simulink model "LKARefMdl"  (R2025b)
settings: Solver=FixedStepDiscrete  StartTime=0.0  StopTime=inf  FixedStep=Ts  RelTol=1e-3
values from neighbouring files (symbols this model uses):
  PredictionHorizon = 30    [helperLKASetUp.m]
  Ts = 0.1/2    (= 0.05)    [helperLKASetUp.m]
libraries: simulink x4, simulink_extras x1, mpcadaslib x1
settings Model: Creator=The MathWorks, Inc.  LastModifiedBy=diogo
settings SolverCC: AlgebraicLoopSolver=TrustRegion
settings DataIOCC: SaveOutput=off  SaveTime=off  ReturnWorkspaceOutputs=off
settings OptimizationCC: DefaultParameterBehavior=Inlined  UseFloatMulNetSlope=on  DefaultUnderspecifiedDataType=single  UseSpecifiedMinMax=on  InlineInvariantSignals=on  EnhancedBackFolding=on  StrengthReduction=on  PassReuseOutputArgsAs=Individual arguments  ZeroExternalMemoryAtStartup=off  ZeroInternalMemoryAtStartup=off  NoFixptDivByZeroProtection=on  EfficientFloat2IntCast=on  OptimizeBlockOrder=speed  DifferentSizesBufferReuse=on  EfficientTunableParamExpr=on
settings DebuggingCC: ParameterPrecisionLossMsg=none  ParameterTunabilityLossMsg=error  UnconnectedInputMsg=warning  UnconnectedOutputMsg=warning  UnconnectedLineMsg=warning  ArithmeticOperatorsInVariantConditions=warning
settings HardwareCC: ProdLongLongMode=on
settings ModelReferenceCC: EnableRefExpFcnMdlSchedulingChecks=on
settings SFSimCC: SimUseLocalCustomCode=off  MATLABDynamicMemAlloc=off  CustomCodeUndefinedFunction=UseInterfaceOnly  SimTargetLang=C++  SimDLTargetLibrary=mkl-dnn
settings RTWCC: SystemTargetFile=ert.tlc  TemplateMakefile=ert_default_tmf  GenerateReport=on  RTWUseLocalCustomCode=off  BuildConfiguration=Faster Runs  IncludeHyperlinkInReport=on  LaunchReport=on  TargetLang=C++  GenerateTraceInfo=on  GenerateTraceReport=on  GenerateTraceReportSl=on  GenerateTraceReportSf=on  GenerateTraceReportEml=on  GPUComputeCapability=3.5  DLArmComputeVersion=19.05  Description=Embedded Coder
settings CodeAppCC: ForceParamTrailComments=on  IgnoreCustomStorageClasses=off  OperatorAnnotations=on  SimulinkDataObjDesc=on  SFDataObjDesc=on  InsertBlockDesc=on
settings ERTTargetCC: RootIOFormat=Structure reference  ERTCustomFileTemplate=example_file_process.tlc  DynamicArrayContainerType=coder::array  TargetLangStandard=C++03 (ISO)  GenerateSampleERTMain=on  CombineSignalStateStructs=on  SuppressErrorStatus=on  CodeInterfacePackaging=C++ class  SubcomponentCodeInterfacePackaging=C++ class

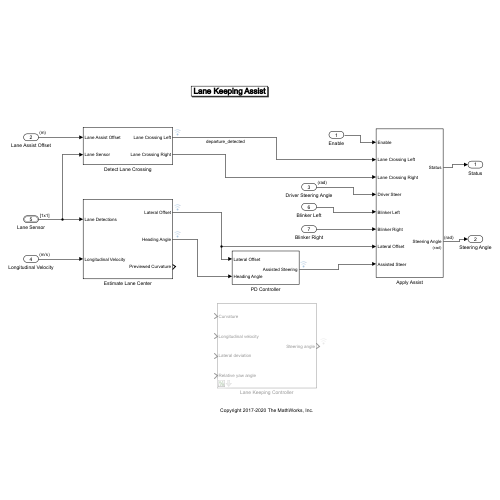
[thumbnail: Simulink's stored preview of the top-level diagram]
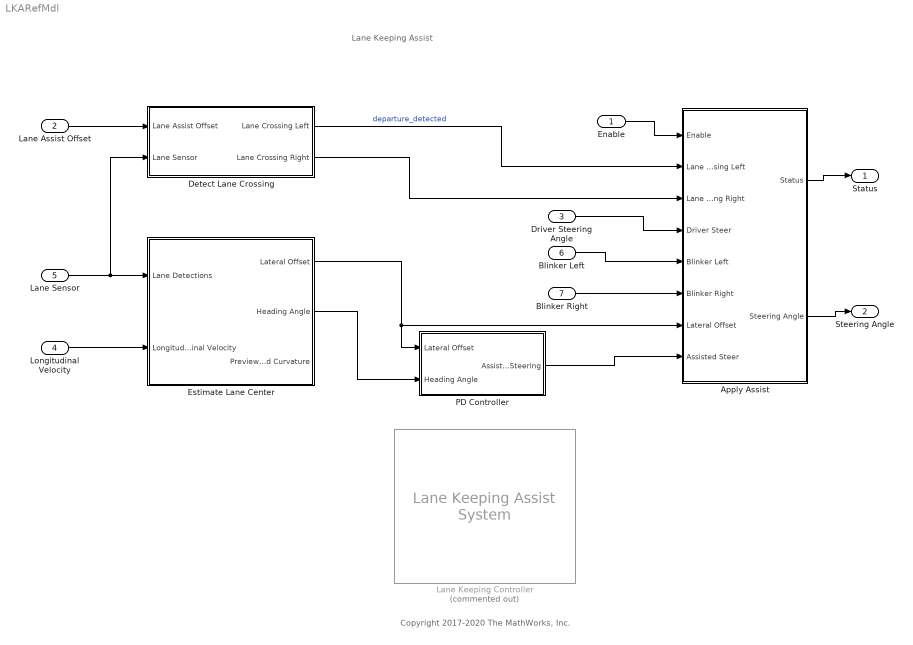
== system LKARefMdl ==
  note: Copyright 2017-2020 The MathWorks, Inc.
  note: Lane Keeping Assist
  Enable : Inport  OutDataTypeStr=boolean  SampleTime=Ts
  Lane Assist Offset : Inport  Port=2  OutDataTypeStr=single  Unit=m  SampleTime=Ts
  Driver Steering Angle : Inport  Port=3  Unit=rad
  Longitudinal Velocity : Inport  Port=4  OutDataTypeStr=single  Unit=m/s  SampleTime=Ts
  Lane Sensor : Inport  Port=5  OutDataTypeStr=Bus: LaneSensor  PortDimensions=[1 1]  SampleTime=Ts  BusOutputAsStruct=on
  Blinker Left : Inport  Port=6
  Blinker Right : Inport  Port=7
  Apply Assist : Subsystem
  Detect Lane Crossing : Subsystem
  Estimate Lane Center : Subsystem  VariantControl=v2
  Lane Keeping Controller : mpcadaslib/Lane Keeping Assist System  Commented=on  ModelType=Use vehicle parameters  VehicleMass=m  VehicleYawInertia=Iz  LengthToFront=lf  LengthToRear=lr  FrontTireStiffness=Cf  RearTireStiffness=Cr  EgoModelMatrixA=[-4.4021 ,-12.4603;1.3913,-5.1868]  EgoModelMatrixB=[24.1270;15.8609]  EgoModelMatrixC=[1,0;0,1]  InitialLongVel=v0_ego  TransportLag=0  MinSteering=-0.5  umin_ext=off  MaxSteering=0.5  umax_ext=off  Ts=Ts  PredictionHorizon=PredictionHorizon  ControllerBehavior=0.200  suboptimal=off  maxiter=10  datatypeopt=single  optmode=off  trackmode=off
  PD Controller : Subsystem
  Status : Outport  PortDimensions=1  VectorParamsAs1DForOutWhenUnconnected=off
  Steering Angle : Outport  Port=2  PortDimensions=1  VectorParamsAs1DForOutWhenUnconnected=off
  wires:
  Lane Assist Offset/1 -> Detect Lane Crossing/1(Lane Assist Offset)
  Driver Steering Angle/1 -> Apply Assist/4(Driver Steer)
  Enable/1 -> Apply Assist/1(Enable)
  Apply Assist/1(Status) -> Status/1
  Apply Assist/2(Steering Angle) -> Steering Angle/1
  Detect Lane Crossing/1(Lane Crossing Left) -> Apply Assist/2(Lane Crossing Left)  "departure_detected"
  Longitudinal Velocity/1 -> Estimate Lane Center/2(Longitudinal Velocity)
  Lane Sensor/1 -> Detect Lane Crossing/2(Lane Sensor), Estimate Lane Center/1(Lane Detections)
  Estimate Lane Center/1(Lateral Offset) -> PD Controller/1(Lateral Offset), Apply Assist/7(Lateral Offset)
  Estimate Lane Center/2(Heading Angle) -> PD Controller/2(Heading Angle)
  PD Controller/1(Assisted Steering) -> Apply Assist/8(Assisted Steer)
  Blinker Left/1 -> Apply Assist/5(Blinker Left)
  Detect Lane Crossing/2(Lane Crossing Right) -> Apply Assist/3(Lane Crossing Right)
  Blinker Right/1 -> Apply Assist/6(Blinker Right)

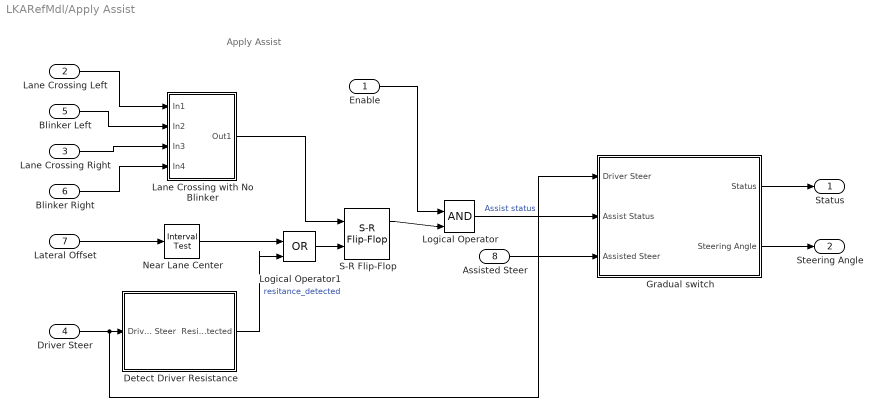
== system LKARefMdl/Apply Assist ==
  note: Apply Assist
  Enable : Inport
  Lane Crossing Left : Inport  Port=2
  Lane Crossing Right : Inport  Port=3
  Driver Steer : Inport  Port=4
  Blinker Left : Inport  Port=5
  Blinker Right : Inport  Port=6
  Lateral Offset : Inport  Port=7
  Assisted Steer : Inport  Port=8
  "Detect Driver Resistance " : Subsystem
  Gradual switch : Subsystem
  Lane Crossing with No Blinker : Subsystem
  Logical Operator : Logic  IconShape=distinctive  AllPortsSameDT=off  OutDataTypeStr=boolean
  Logical Operator1 : Logic  Operator=OR  IconShape=distinctive  AllPortsSameDT=off  OutDataTypeStr=boolean
  Near Lane Center : simulink/Logic and Bit Operations/Interval Test  IntervalClosedRight=on  uplimit=0.1  IntervalClosedLeft=on  lowlimit=-0.1  OutDataTypeStr=boolean
  S-R Flip-Flop : simulink_extras/Flip Flops/S-R Flip-Flop  initial_condition=0
  Status : Outport  VectorParamsAs1DForOutWhenUnconnected=off
  Steering Angle : Outport  Port=2  Unit=rad  VectorParamsAs1DForOutWhenUnconnected=off
  wires:
  Enable/1 -> Logical Operator/1
  Logical Operator/1 -> Gradual switch/2(Assist Status)  "Assist status"
  Driver Steer/1 -> "Detect Driver Resistance "/1(Driver Steer), Gradual switch/1(Driver Steer)
  Gradual switch/1(Status) -> Status/1
  Gradual switch/2(Steering Angle) -> Steering Angle/1
  S-R Flip-Flop/1 -> Logical Operator/2
  Lane Crossing Left/1 -> Lane Crossing with No Blinker/1(In1)
  Blinker Left/1 -> Lane Crossing with No Blinker/2(In2)
  Lane Crossing Right/1 -> Lane Crossing with No Blinker/3(In3)
  Blinker Right/1 -> Lane Crossing with No Blinker/4(In4)
  Lane Crossing with No Blinker/1(Out1) -> S-R Flip-Flop/1
  Near Lane Center/1 -> Logical Operator1/1
  Lateral Offset/1 -> Near Lane Center/1
  "Detect Driver Resistance "/1(Resistance Detected) -> Logical Operator1/2  "resitance_detected"
  Logical Operator1/1 -> S-R Flip-Flop/2
  Assisted Steer/1 -> Gradual switch/3(Assisted Steer)

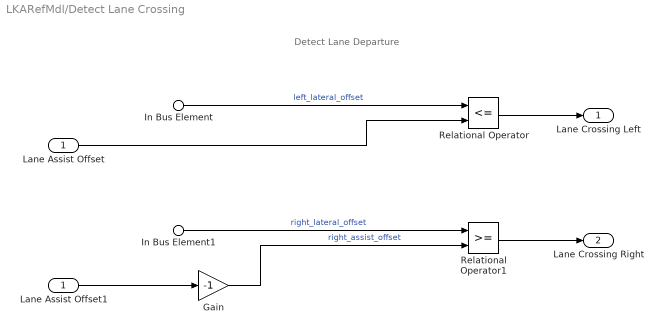
== system LKARefMdl/Detect Lane Crossing ==
  note: Detect Lane Departure
  Lane Assist Offset : Inport
  In Bus Element : Inport  Port=2  PortName=Lane Sensor  Element=Left.LateralOffset
  In Bus Element1 : Inport  Port=2  PortName=Lane Sensor  Element=Right.LateralOffset
  Gain : Gain  Gain=-1
  Lane Assist Offset1 : InportShadow
  Relational Operator : RelationalOperator  Operator=<=  OutDataTypeStr=boolean  RndMeth=Simplest  InputSameDT=off
  Relational Operator1 : RelationalOperator  OutDataTypeStr=boolean  RndMeth=Simplest  InputSameDT=off
  Lane Crossing Left : Outport  VectorParamsAs1DForOutWhenUnconnected=off
  Lane Crossing Right : Outport  Port=2  VectorParamsAs1DForOutWhenUnconnected=off
  wires:
  Lane Assist Offset/1 -> Relational Operator/2
  In Bus Element/1 -> Relational Operator/1  "left_lateral_offset"
  Lane Assist Offset1/1 -> Gain/1
  In Bus Element1/1 -> Relational Operator1/1  "right_lateral_offset"
  Gain/1 -> Relational Operator1/2  "right_assist_offset"
  Relational Operator1/1 -> Lane Crossing Right/1
  Relational Operator/1 -> Lane Crossing Left/1

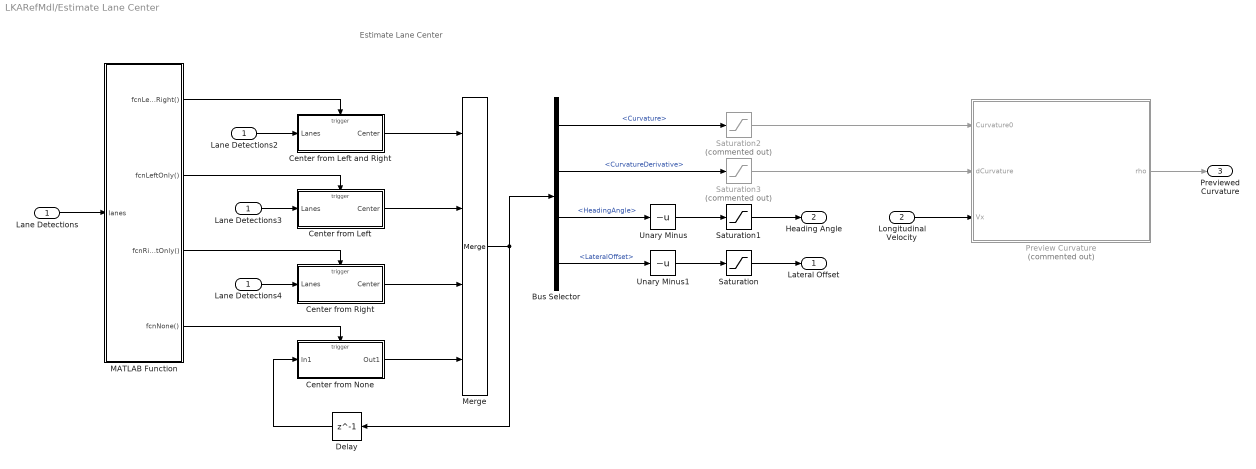
== system LKARefMdl/Estimate Lane Center ==
  note: Estimate Lane Center
  Lane Detections : Inport
  Longitudinal Velocity : Inport  Port=2  OutDataTypeStr=single
  Bus Selector : BusSelector  OutputSignals=Curvature,CurvatureDerivative,HeadingAngle,LateralOffset
  Center from Left : Subsystem  TreatAsAtomicUnit=on
  Center from Left and Right : Subsystem  TreatAsAtomicUnit=on
  Center from None : Subsystem  TreatAsAtomicUnit=on
  Center from Right : Subsystem  TreatAsAtomicUnit=on
  Delay : Delay  DelayLength=1
  Lane Detections2 : InportShadow
  Lane Detections3 : InportShadow
  Lane Detections4 : InportShadow
  MATLAB Function : MATLAB Function  TreatAsAtomicUnit=on
  Merge : Merge  Inputs=4
  Preview Curvature : MATLAB Function  Commented=on  TreatAsAtomicUnit=on  SystemSampleTime=Ts
  Saturation : Saturate
  Saturation1 : Saturate  UpperLimit=0.6  LowerLimit=-0.6
  Saturation2 : Saturate  Commented=on  UpperLimit=0.15  LowerLimit=-0.15
  Saturation3 : Saturate  Commented=on  UpperLimit=0.06  LowerLimit=-0.06
  Unary Minus : UnaryMinus
  Unary Minus1 : UnaryMinus
  Lateral Offset : Outport  VectorParamsAs1DForOutWhenUnconnected=off
  Heading Angle : Outport  Port=2  VectorParamsAs1DForOutWhenUnconnected=off
  Previewed Curvature : Outport  Port=3  VectorParamsAs1DForOutWhenUnconnected=off
  wires:
  Bus Selector/3 -> Unary Minus/1  "<HeadingAngle>"
  Bus Selector/4 -> Unary Minus1/1  "<LateralOffset>"
  Unary Minus1/1 -> Saturation/1
  Longitudinal Velocity/1 -> Preview Curvature/3(Vx)
  Unary Minus/1 -> Saturation1/1
  Saturation/1 -> Lateral Offset/1
  Saturation1/1 -> Heading Angle/1
  Merge/1 -> Delay/1, Bus Selector/1
  Center from Left/1(Center) -> Merge/2
  MATLAB Function/4(fcnNone()) -> Center from None/Trigger
  MATLAB Function/3(fcnRightOnly()) -> Center from Right/Trigger
  Lane Detections2/1 -> Center from Left and Right/1(Lanes)
  Lane Detections/1 -> MATLAB Function/1(lanes)
  Center from Left and Right/1(Center) -> Merge/1
  Delay/1 -> Center from None/1(In1)
  MATLAB Function/1(fcnLeftAndRight()) -> Center from Left and Right/Trigger
  Center from None/1(Out1) -> Merge/4
  MATLAB Function/2(fcnLeftOnly()) -> Center from Left/Trigger
  Lane Detections4/1 -> Center from Right/1(Lanes)
  Lane Detections3/1 -> Center from Left/1(Lanes)
  Center from Right/1(Center) -> Merge/3
  Bus Selector/2 -> Saturation3/1  "<CurvatureDerivative>"
  Preview Curvature/1(rho) -> Previewed Curvature/1
  Saturation3/1 -> Preview Curvature/2(dCurvature)
  Saturation2/1 -> Preview Curvature/1(Curvature0)
  Bus Selector/1 -> Saturation2/1  "<Curvature>"

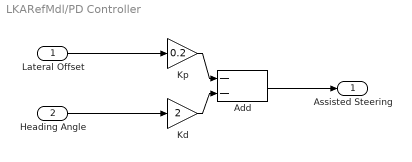
== system LKARefMdl/PD Controller ==
  Lateral Offset : Inport
  Heading Angle : Inport  Port=2
  Add : Sum  Inputs=--
  Kd : Gain  Gain=2
  Kp : Gain  Gain=0.2
  Assisted Steering : Outport
  wires:
  Kp/1 -> Add/1
  Add/1 -> Assisted Steering/1
  Kd/1 -> Add/2
  Heading Angle/1 -> Kd/1
  Lateral Offset/1 -> Kp/1

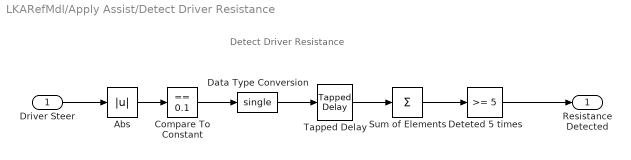
== system LKARefMdl/Apply Assist/Detect Driver Resistance  ==
  note: Detect Driver Resistance
  Driver Steer : Inport
  Abs : Abs  SaturateOnIntegerOverflow=off
  Compare To Constant : simulink/Logic and Bit Operations/Compare To Constant  relop===  const=0.1  OutDataTypeStr=boolean
  Data Type Conversion : DataTypeConversion  OutDataTypeStr=single  SaturateOnIntegerOverflow=off  RndMeth=Floor
  Deteted 5 times : simulink/Logic and Bit Operations/Compare To Constant  relop=>=  const=5  OutDataTypeStr=boolean
  Sum of Elements : Sum  Inputs=+
  Tapped Delay : simulink/Discrete/Tapped Delay  vinit=0.0  samptime=-1  NumDelays=5  DelayOrder=Oldest  includeCurrent=off
  Resistance Detected : Outport  VectorParamsAs1DForOutWhenUnconnected=off
  wires:
  Driver Steer/1 -> Abs/1
  Deteted 5 times/1 -> Resistance Detected/1
  Data Type Conversion/1 -> Tapped Delay/1
  Tapped Delay/1 -> Sum of Elements/1
  Sum of Elements/1 -> Deteted 5 times/1
  Abs/1 -> Compare To Constant/1
  Compare To Constant/1 -> Data Type Conversion/1

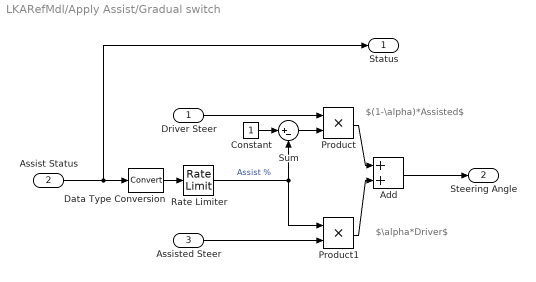
== system LKARefMdl/Apply Assist/Gradual switch ==
  note: $\alpha*Driver$
  note: $(1-\alpha)*Assisted$
  Driver Steer : Inport
  Assist Status : Inport  Port=2
  Assisted Steer : Inport  Port=3
  Add : Sum
  Constant : Constant
  Data Type Conversion : DataTypeConversion  SaturateOnIntegerOverflow=off  RndMeth=Floor
  Product : Product
  Product1 : Product
  Rate Limiter : RateLimiter  RisingSlewLimit=0.25  FallingSlewLimit=-0.25  SampleTimeMode=inherited
  Sum : Sum  Inputs=|+-
  Status : Outport  VectorParamsAs1DForOutWhenUnconnected=off
  Steering Angle : Outport  Port=2  Unit=rad  VectorParamsAs1DForOutWhenUnconnected=off
  wires:
  Rate Limiter/1 -> Product1/1, Sum/2  "Assist %"
  Product/1 -> Add/1
  Assist Status/1 -> Status/1, Data Type Conversion/1
  Constant/1 -> Sum/1
  Add/1 -> Steering Angle/1
  Sum/1 -> Product/2
  Assisted Steer/1 -> Product1/2
  Product1/1 -> Add/2
  Driver Steer/1 -> Product/1
  Data Type Conversion/1 -> Rate Limiter/1

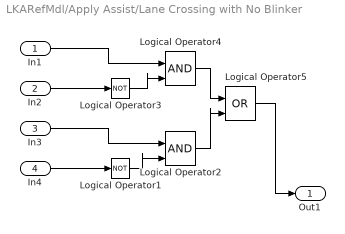
== system LKARefMdl/Apply Assist/Lane Crossing with No Blinker ==
  In1 : Inport
  In2 : Inport  Port=2
  In3 : Inport  Port=3
  In4 : Inport  Port=4
  Logical Operator1 : Logic  Operator=NOT  IconShape=distinctive  AllPortsSameDT=off  OutDataTypeStr=boolean
  Logical Operator2 : Logic  IconShape=distinctive  AllPortsSameDT=off  OutDataTypeStr=boolean
  Logical Operator3 : Logic  Operator=NOT  IconShape=distinctive  AllPortsSameDT=off  OutDataTypeStr=boolean
  Logical Operator4 : Logic  IconShape=distinctive  AllPortsSameDT=off  OutDataTypeStr=boolean
  Logical Operator5 : Logic  Operator=OR  IconShape=distinctive  AllPortsSameDT=off  OutDataTypeStr=boolean
  Out1 : Outport
  wires:
  Logical Operator4/1 -> Logical Operator5/1
  Logical Operator2/1 -> Logical Operator5/2
  Logical Operator3/1 -> Logical Operator4/2
  In2/1 -> Logical Operator3/1
  Logical Operator5/1 -> Out1/1
  In4/1 -> Logical Operator1/1
  Logical Operator1/1 -> Logical Operator2/2
  In3/1 -> Logical Operator2/1
  In1/1 -> Logical Operator4/1

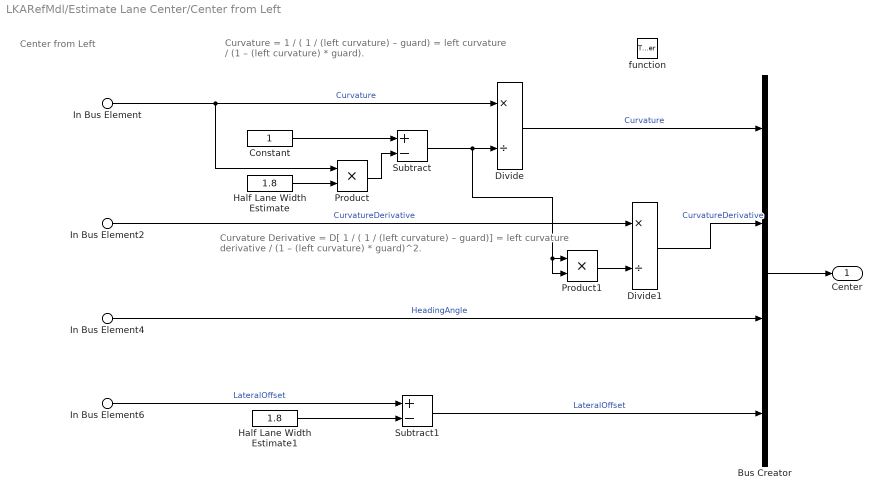
== system LKARefMdl/Estimate Lane Center/Center from Left ==
  note: Curvature
      | = 1 / ( 1 / (left curvature) – guard)
      | = left curvature / (1 – (left curvature) * guard).
  note: Center from Left
  note: Curvature Derivative
      | = D[ 1 / ( 1 / (left curvature) – guard)]
      | = left curvature derivative / (1 – (left curvature) * guard)^2.
  In Bus Element : Inport  PortName=Lanes  Element=Left.Curvature
  In Bus Element2 : Inport  PortName=Lanes  Element=Left.CurvatureDerivative
  In Bus Element4 : Inport  PortName=Lanes  Element=Left.HeadingAngle
  In Bus Element6 : Inport  PortName=Lanes  Element=Left.LateralOffset
  function : TriggerPort  TriggerType=function-call  VariantControl=Variant
  Bus Creator : BusCreator  Inputs=4
  Constant : Constant  OutDataTypeStr=Inherit: Inherit via back propagation
  Divide : Product  Inputs=*/
  Divide1 : Product  Inputs=*/
  Half Lane Width Estimate : Constant  Value=1.8  OutDataTypeStr=Inherit: Inherit via back propagation
  Half Lane Width Estimate1 : Constant  Value=1.8  OutDataTypeStr=Inherit: Inherit via back propagation
  Product : Product
  Product1 : Product
  Subtract : Sum  Inputs=+-
  Subtract1 : Sum  Inputs=+-
  Center : Outport  VectorParamsAs1DForOutWhenUnconnected=off
  wires:
  Bus Creator/1 -> Center/1
  Divide1/1 -> Bus Creator/2  "CurvatureDerivative"
  Divide/1 -> Bus Creator/1  "Curvature"
  In Bus Element4/1 -> Bus Creator/3  "HeadingAngle"
  Subtract1/1 -> Bus Creator/4  "LateralOffset"
  In Bus Element/1 -> Product/1, Divide/1  "Curvature"
  Subtract/1 -> Product1/2, Product1/1, Divide/2
  Half Lane Width Estimate/1 -> Product/2
  Constant/1 -> Subtract/1
  In Bus Element2/1 -> Divide1/1  "CurvatureDerivative"
  Product1/1 -> Divide1/2
  In Bus Element6/1 -> Subtract1/1  "LateralOffset"
  Half Lane Width Estimate1/1 -> Subtract1/2
  Product/1 -> Subtract/2

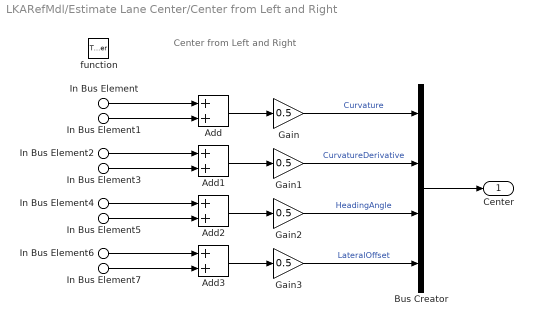
== system LKARefMdl/Estimate Lane Center/Center from Left and Right ==
  note: Center from Left and Right
  In Bus Element : Inport  PortName=Lanes  Element=Left.Curvature
  In Bus Element2 : Inport  PortName=Lanes  Element=Left.CurvatureDerivative
  In Bus Element4 : Inport  PortName=Lanes  Element=Left.HeadingAngle
  In Bus Element6 : Inport  PortName=Lanes  Element=Left.LateralOffset
  In Bus Element1 : Inport  PortName=Lanes  Element=Right.Curvature
  In Bus Element3 : Inport  PortName=Lanes  Element=Right.CurvatureDerivative
  In Bus Element5 : Inport  PortName=Lanes  Element=Right.HeadingAngle
  In Bus Element7 : Inport  PortName=Lanes  Element=Right.LateralOffset
  function : TriggerPort  TriggerType=function-call  VariantControl=Variant
  Add{,1..3} (4 alike) : Sum
  Bus Creator : BusCreator  Inputs=4
  Gain{,1..3} (4 alike) : Gain  Gain=0.5
  Center : Outport  VectorParamsAs1DForOutWhenUnconnected=off
  wires:
  Add/1 -> Gain/1
  Gain/1 -> Bus Creator/1  "Curvature"
  Add1/1 -> Gain1/1
  Gain1/1 -> Bus Creator/2  "CurvatureDerivative"
  Add2/1 -> Gain2/1
  Gain2/1 -> Bus Creator/3  "HeadingAngle"
  Add3/1 -> Gain3/1
  Gain3/1 -> Bus Creator/4  "LateralOffset"
  Bus Creator/1 -> Center/1
  In Bus Element/1 -> Add/1
  In Bus Element1/1 -> Add/2
  In Bus Element2/1 -> Add1/1
  In Bus Element3/1 -> Add1/2
  In Bus Element4/1 -> Add2/1
  In Bus Element5/1 -> Add2/2
  In Bus Element7/1 -> Add3/2
  In Bus Element6/1 -> Add3/1

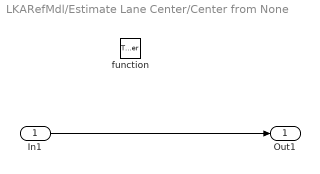
== system LKARefMdl/Estimate Lane Center/Center from None ==
  In1 : Inport
  function : TriggerPort  TriggerType=function-call  VariantControl=Variant
  Out1 : Outport  VectorParamsAs1DForOutWhenUnconnected=off
  wires:
  In1/1 -> Out1/1

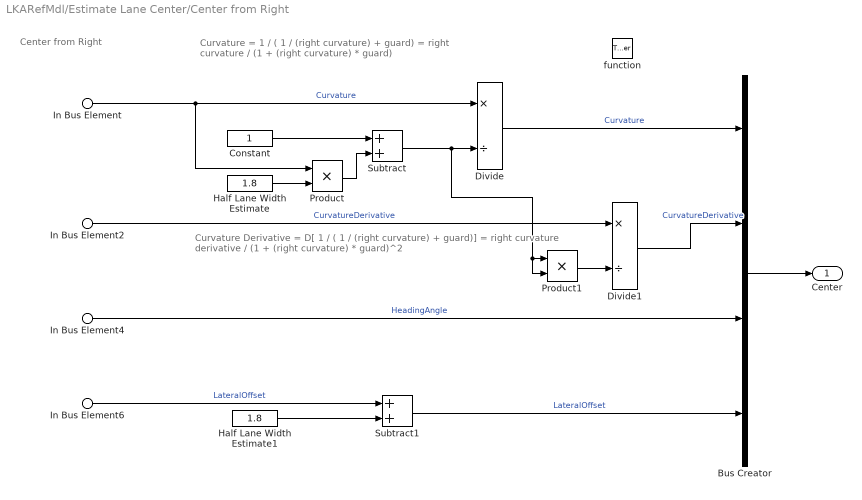
== system LKARefMdl/Estimate Lane Center/Center from Right ==
  note: Center from Right
  note: Curvature
      | = 1 / ( 1 / (right curvature) + guard)
      | = right curvature / (1 + (right curvature) * guard)
  note: Curvature Derivative
      | = D[ 1 / ( 1 / (right curvature) + guard)]
      | = right curvature derivative / (1 + (right curvature) * guard)^2
  In Bus Element : Inport  PortName=Lanes  Element=Right.Curvature
  In Bus Element2 : Inport  PortName=Lanes  Element=Right.CurvatureDerivative
  In Bus Element4 : Inport  PortName=Lanes  Element=Right.HeadingAngle
  In Bus Element6 : Inport  PortName=Lanes  Element=Right.LateralOffset
  function : TriggerPort  TriggerType=function-call  VariantControl=Variant
  Bus Creator : BusCreator  Inputs=4
  Constant : Constant  OutDataTypeStr=Inherit: Inherit via back propagation
  Divide : Product  Inputs=*/
  Divide1 : Product  Inputs=*/
  Half Lane Width Estimate : Constant  Value=1.8  OutDataTypeStr=Inherit: Inherit via back propagation
  Half Lane Width Estimate1 : Constant  Value=1.8  OutDataTypeStr=Inherit: Inherit via back propagation
  Product : Product
  Product1 : Product
  Subtract : Sum
  Subtract1 : Sum
  Center : Outport  VectorParamsAs1DForOutWhenUnconnected=off
  wires:
  In Bus Element2/1 -> Divide1/1  "CurvatureDerivative"
  Divide1/1 -> Bus Creator/2  "CurvatureDerivative"
  Product1/1 -> Divide1/2
  In Bus Element4/1 -> Bus Creator/3  "HeadingAngle"
  Half Lane Width Estimate1/1 -> Subtract1/2
  In Bus Element6/1 -> Subtract1/1  "LateralOffset"
  Divide/1 -> Bus Creator/1  "Curvature"
  Subtract1/1 -> Bus Creator/4  "LateralOffset"
  Bus Creator/1 -> Center/1
  In Bus Element/1 -> Product/1, Divide/1  "Curvature"
  Subtract/1 -> Product1/2, Product1/1, Divide/2
  Constant/1 -> Subtract/1
  Product/1 -> Subtract/2
  Half Lane Width Estimate/1 -> Product/2

== matlab function LKARefMdl/Estimate Lane Center/MATLAB Function ==
  data: lanes input
  events: fcnLeftAndRight output FUNCTION_CALL_EVENT; fcnLeftOnly output FUNCTION_CALL_EVENT; fcnRightOnly output FUNCTION_CALL_EVENT; fcnNone output FUNCTION_CALL_EVENT
function fcn(lanes)

leftStrength  = lanes.Left.Strength;
rightStrength = lanes.Right.Strength;

if (leftStrength > 0) && (rightStrength > 0)
   fcnLeftAndRight();
   
elseif leftStrength > 0
    fcnLeftOnly();
    
elseif rightStrength > 0
    fcnRightOnly();
    
else
    fcnNone();
end

== matlab function LKARefMdl/Estimate Lane Center/Preview Curvature ==
  data: rho output; Curvature0 input; dCurvature input; Vx input; Ts parameter; PredictionHorizon parameter
function rho = predictCurvature(Curvature0,dCurvature,Vx, Ts, PredictionHorizon)
% Curvature0 = initial curvature per unit length                  [1/m]
% dCurvature = (constant) derivative of curvature per unit length [1/m^2]
% CurvatureLength = length for which the clothoid model is valid [m]
% Vx = speed of vehicle

% We want to export a set of curvatures at a uniform sample time ahead.
% t is this vector which goes up to 1 second in the future or having
% enough time to reach the known length in curvature (whichever is smaller)

% To enable truncation by curvelength, mark output "rho" as varsize
%t = 0:Ts:min(1,CurvatureLength/Vx);

t = zeros(PredictionHorizon+1,1);
for i=1:numel(t)
    t(i) = (i-1).*Ts;
end

% We compute the curvature vector rho(t) using the specified clothoid model
rho = Curvature0 + dCurvature*Vx*t;
